simulink model "pendulum_demo"  (R2015a)
settings: Solver=ode45  SolverMode=SingleTasking  StartTime=0  StopTime=15  RelTol=1e-3  AbsTol=1e-6
PreLoadFcn:
  | load pendulum_demo
model workspace (MAT data in the model file):
  pendulum_optim = sldodialogs.data.SessionData
  pendulum_optim.Version = '3.0'
  pendulum_optim.Data.ModelName = 'pendulum_demo'
  pendulum_optim.Data.ToolData.ResponseOptimization.Options = sdo.OptimizeOptions
  pendulum_optim.Data.ToolData.ResponseOptimization.Options.Method = 'fminsearch'
  pendulum_optim.Data.ToolData.ResponseOptimization.Options.MethodOptions.Display = 'iter'
  pendulum_optim.Data.ToolData.ResponseOptimization.Options.MethodOptions.MaxFunEvals = 99
  pendulum_optim.Data.ToolData.ResponseOptimization.Options.MethodOptions.MaxIter = 49
  pendulum_optim.Data.ToolData.ResponseOptimization.Options.MethodOptions.TolFun = 0.001
  pendulum_optim.Data.ToolData.ResponseOptimization.Options.MethodOptions.TolX = 0.001
  pendulum_optim.Data.ToolData.ResponseOptimization.Options.MethodOptions.FunValCheck = 'off'
  pendulum_optim.Data.ToolData.ResponseOptimization.Options.MethodOptions.OutputFcn = []
  pendulum_optim.Data.ToolData.ResponseOptimization.Options.MethodOptions.PlotFcns = []
  pendulum_optim.Data.ToolData.ResponseOptimization.Options.MethodOptions.ActiveConstrTol = []
  pendulum_optim.Data.ToolData.ResponseOptimization.Options.MethodOptions.Algorithm = []
  pendulum_optim.Data.ToolData.ResponseOptimization.Options.MethodOptions.AlwaysHonorConstraints = []
  pendulum_optim.Data.ToolData.ResponseOptimization.Options.MethodOptions.BranchStrategy = []
  pendulum_optim.Data.ToolData.ResponseOptimization.Options.MethodOptions.DerivativeCheck = []
  pendulum_optim.Data.ToolData.ResponseOptimization.Options.MethodOptions.Diagnostics = []
  pendulum_optim.Data.ToolData.ResponseOptimization.Options.MethodOptions.DiffMaxChange = []
  pendulum_optim.Data.ToolData.ResponseOptimization.Options.MethodOptions.DiffMinChange = []
  pendulum_optim.Data.ToolData.ResponseOptimization.Options.MethodOptions.FinDiffRelStep = []
  pendulum_optim.Data.ToolData.ResponseOptimization.Options.MethodOptions.FinDiffType = []
  pendulum_optim.Data.ToolData.ResponseOptimization.Options.MethodOptions.GoalsExactAchieve = []
  pendulum_optim.Data.ToolData.ResponseOptimization.Options.MethodOptions.GradConstr = []
  pendulum_optim.Data.ToolData.ResponseOptimization.Options.MethodOptions.GradObj = []
  pendulum_optim.Data.ToolData.ResponseOptimization.Options.MethodOptions.HessFcn = []
  pendulum_optim.Data.ToolData.ResponseOptimization.Options.MethodOptions.Hessian = []
  pendulum_optim.Data.ToolData.ResponseOptimization.Options.MethodOptions.HessMult = []
  pendulum_optim.Data.ToolData.ResponseOptimization.Options.MethodOptions.HessPattern = []
  pendulum_optim.Data.ToolData.ResponseOptimization.Options.MethodOptions.HessUpdate = []
  pendulum_optim.Data.ToolData.ResponseOptimization.Options.MethodOptions.InitialHessType = []
  pendulum_optim.Data.ToolData.ResponseOptimization.Options.MethodOptions.InitialHessMatrix = []
  pendulum_optim.Data.ToolData.ResponseOptimization.Options.MethodOptions.InitBarrierParam = []
  pendulum_optim.Data.ToolData.ResponseOptimization.Options.MethodOptions.InitTrustRegionRadius = []
  pendulum_optim.Data.ToolData.ResponseOptimization.Options.MethodOptions.Jacobian = []
  pendulum_optim.Data.ToolData.ResponseOptimization.Options.MethodOptions.JacobMult = []
  pendulum_optim.Data.ToolData.ResponseOptimization.Options.MethodOptions.JacobPattern = []
  pendulum_optim.Data.ToolData.ResponseOptimization.Options.MethodOptions.LargeScale = []
  pendulum_optim.Data.ToolData.ResponseOptimization.Options.MethodOptions.LineSearchType = []
  pendulum_optim.Data.ToolData.ResponseOptimization.Options.MethodOptions.MaxNodes = []
  pendulum_optim.Data.ToolData.ResponseOptimization.Options.MethodOptions.MaxPCGIter = []
  pendulum_optim.Data.ToolData.ResponseOptimization.Options.MethodOptions.MaxProjCGIter = []
  pendulum_optim.Data.ToolData.ResponseOptimization.Options.MethodOptions.MaxRLPIter = []
  pendulum_optim.Data.ToolData.ResponseOptimization.Options.MethodOptions.MaxSQPIter = []
  pendulum_optim.Data.ToolData.ResponseOptimization.Options.MethodOptions.MaxTime = []
  pendulum_optim.Data.ToolData.ResponseOptimization.Options.MethodOptions.MeritFunction = []
  pendulum_optim.Data.ToolData.ResponseOptimization.Options.MethodOptions.MinAbsMax = []
  pendulum_optim.Data.ToolData.ResponseOptimization.Options.MethodOptions.NodeDisplayInterval = []
  pendulum_optim.Data.ToolData.ResponseOptimization.Options.MethodOptions.NodeSearchStrategy = []
  pendulum_optim.Data.ToolData.ResponseOptimization.Options.MethodOptions.NoStopIfFlatInfeas = []
  pendulum_optim.Data.ToolData.ResponseOptimization.Options.MethodOptions.ObjectiveLimit = []
  pendulum_optim.Data.ToolData.ResponseOptimization.Options.MethodOptions.PhaseOneTotalScaling = []
  pendulum_optim.Data.ToolData.ResponseOptimization.Options.MethodOptions.Preconditioner = []
  pendulum_optim.Data.ToolData.ResponseOptimization.Options.MethodOptions.PrecondBandWidth = []
  pendulum_optim.Data.ToolData.ResponseOptimization.Options.MethodOptions.RelLineSrchBnd = []
  pendulum_optim.Data.ToolData.ResponseOptimization.Options.MethodOptions.RelLineSrchBndDuration = []
  pendulum_optim.Data.ToolData.ResponseOptimization.Options.MethodOptions.ScaleProblem = []
  pendulum_optim.Data.ToolData.ResponseOptimization.Options.MethodOptions.Simplex = []
  pendulum_optim.Data.ToolData.ResponseOptimization.Options.MethodOptions.SubproblemAlgorithm = []
  pendulum_optim.Data.ToolData.ResponseOptimization.Options.MethodOptions.TolCon = 0.001
  pendulum_optim.Data.ToolData.ResponseOptimization.Options.MethodOptions.TolConSQP = []
  pendulum_optim.Data.ToolData.ResponseOptimization.Options.MethodOptions.TolGradCon = []
  pendulum_optim.Data.ToolData.ResponseOptimization.Options.MethodOptions.TolPCG = []
  pendulum_optim.Data.ToolData.ResponseOptimization.Options.MethodOptions.TolProjCG = []
  pendulum_optim.Data.ToolData.ResponseOptimization.Options.MethodOptions.TolProjCGAbs = []
  pendulum_optim.Data.ToolData.ResponseOptimization.Options.MethodOptions.TolRLPFun = []
  pendulum_optim.Data.ToolData.ResponseOptimization.Options.MethodOptions.TolXInteger = []
  pendulum_optim.Data.ToolData.ResponseOptimization.Options.MethodOptions.TypicalX = []
  pendulum_optim.Data.ToolData.ResponseOptimization.Options.MethodOptions.UseParallel = 'never'
  pendulum_optim.Data.ToolData.ResponseOptimization.DesignVariables = 'DesignVars'
  pendulum_optim.Data.ToolType = 'ResponseOptimization'
  pendulum_optim.Data.Workspace.LocalWorkspace.DesignVars(1) = param.Continuous
  pendulum_optim.Data.Workspace.LocalWorkspace.DesignVars(1).Scale_ = -3
  pendulum_optim.Data.Workspace.LocalWorkspace.DesignVars(1).Size_ = [1 1]
  pendulum_optim.Data.Workspace.LocalWorkspace.DesignVars(1).Value_ = -3
  pendulum_optim.Data.Workspace.LocalWorkspace.DesignVars(1).pID = paramid.Variable
  pendulum_optim.Data.Workspace.LocalWorkspace.DesignVars(1).pID.Name = 'Kf'
  pendulum_optim.Data.Workspace.LocalWorkspace.DesignVars(2) = param.Continuous
  pendulum_optim.Data.Workspace.LocalWorkspace.DesignVars(2).Scale_ = 0
  pendulum_optim.Data.Workspace.LocalWorkspace.DesignVars(2).Size_ = [1 1]
  pendulum_optim.Data.Workspace.LocalWorkspace.DesignVars(2).Value_ = 0
  pendulum_optim.Data.Workspace.LocalWorkspace.DesignVars(2).pID = paramid.Variable
  pendulum_optim.Data.Workspace.LocalWorkspace.DesignVars(2).pID.Name = 'Ki'
  pendulum_optim.Data.Workspace.LocalWorkspace.DesignVars(3) = param.Continuous
  pendulum_optim.Data.Workspace.LocalWorkspace.DesignVars(3).Scale_ = 4.81125224325
  pendulum_optim.Data.Workspace.LocalWorkspace.DesignVars(3).Size_ = [1 1]
  pendulum_optim.Data.Workspace.LocalWorkspace.DesignVars(3).Value_ = 4.81125224325
  pendulum_optim.Data.Workspace.LocalWorkspace.DesignVars(3).pID = paramid.Variable
  pendulum_optim.Data.Workspace.LocalWorkspace.DesignVars(3).pID.Name = 'Kp'
  pendulum_optim.Data.Workspace.HiddenWorkspace = []
undefined symbols (not defined in the file): Kf, Ki, Klqr, Kp
libraries: checkpacklib x2
settings Model: FPTRunName=Active  ExtModeTrigMode=oneshot  Creator=The MathWorks Inc.  LastModifiedBy=Panoply
settings DataIOCC: LimitDataPoints=off  SaveOutput=off  SaveTime=off  SignalLoggingName=logsOut
settings OptimizationCC: BooleanDataType=off  ExpressionDepthLimit=2147483647  InitFltsAndDblsToZero=on  EfficientMapNaN2IntZero=off
settings DebuggingCC: ConsistencyChecking=warning  SaveWithParameterizedLinksMsg=none  UnderspecifiedInitializationDetection=Classic  MergeDetectMultiDrivingBlocksExec=none  CheckExecutionContextPreStartOutputMsg=on  CheckExecutionContextRuntimeOutputMsg=on  SignalResolutionControl=TryResolveAllWithWarning  MultiTaskDSMMsg=warning  MultiTaskCondExecSysMsg=none  FcnCallInpInsideContextMsg=UseLocalSettings  StateNameClashWarn=warning
settings HardwareCC: TargetUnknown=on
settings ModelReferenceCC: UpdateModelReferenceTargets=IfOutOfDate
settings RTWCC: TemplateMakefile=grt_vc.tmf
settings GRTTargetCC: TargetFcnLib=ansi_tfl_tmw.mat  CombineOutputUpdateFcns=off  GRTInterface=on

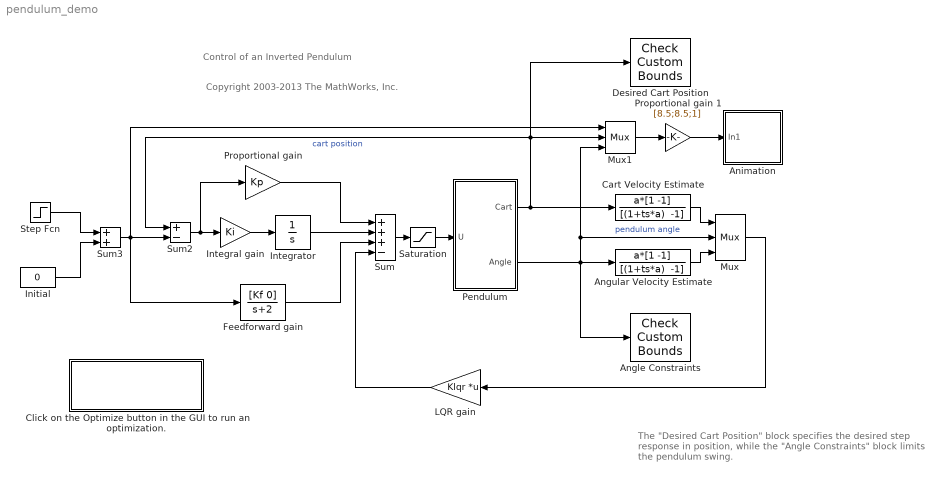
== system pendulum_demo ==
  note: Control of an Inverted Pendulum
  note: The "Desired Cart Position" block specifies the desired
      | step response in position, while the "Angle Constraints"
      | block limits the pendulum swing.
  note: Copyright 2003-2013 The MathWorks, Inc.
  Angle Constraints : checkpacklib/Check Custom Bounds  InstantiateOnLoad=on  enabled=on  stopWhenAssertionFail=off  export=off  ViewDlgPos=[541.717708333334 365.695 504.736979166666 296.7525]  OpenViewOnLoad=off  LaunchViewOnOpen=on  TimeUnits=seconds  EnableUpperBound=on  UpperBoundTimes=[0 15]  UpperBoundAmplitudes=[0.2 0.2]  EnableLowerBound=on  LowerBoundTimes=[0 15]  LowerBoundAmplitudes=[-0.2 -0.2]
  Angular Velocity Estimate : DiscreteTransferFcn  Numerator=a*[1 -1]  Denominator="[(1+ts*a)  -1]"  SampleTime=ts  mask(Finite difference velocity estimator with filter.){hz=10, ts=0.01}
      mask prompts: hz "Cutoff frequency( hz ):"; ts "Sample time:"
      mask help: Finite difference velocity estimator with filter.
      mask init:
      | a=hz*2*pi;
      mask Display: disp('FD w/ filter')
  Animation : Subsystem  mask(Pendulum plot){RefBlock=Initial, doAnimation=false}
      mask prompts: RefBlock "DC reference signal block name:"; doAnimation "Show animation"
      mask help: Pendulum plot
      mask Help: Pendulum animation function using Handle graphics.
      mask Display: plot([-10 10],[0 0],[-2 -2 2 2],[0 1 1 0],[0 3],[1 5])
  Cart Velocity Estimate : DiscreteTransferFcn  Numerator=a*[1 -1]  Denominator="[(1+ts*a)  -1]"  SampleTime=ts  mask(Finite difference velocity estimator with filter.){hz=10, ts=0.01}
      mask prompts: hz "Cutoff frequency( hz ):"; ts "Sample time:"
      mask help: Finite difference velocity estimator with filter.
      mask init:
      | a=hz*2*pi;
      mask Display: disp('FD w/ filter')
  Click on the Optimize button in the GUI to run an optimization. : Subsystem
      settings: OpenFcn=sdotool( slResolve('pendulum_optim', 'pendulum_demo') );
      mask Display: disp('Response Optimization\nGUI with preloaded data')
  Desired Cart Position : checkpacklib/Check Custom Bounds  InstantiateOnLoad=on  enabled=on  stopWhenAssertionFail=off  export=off  ViewDlgPos=[262 234 511 298]  OpenViewOnLoad=on  LaunchViewOnOpen=on  TimeUnits=seconds  EnableUpperBound=on  UpperBoundTimes=[0 6;6 15]  UpperBoundAmplitudes=[1.1 1.1;1.01 1.01]  EnableLowerBound=on  LowerBoundTimes=[0 3;3 6;6 15]  LowerBoundAmplitudes=[-0.1 -0.1;0.882608695652174 0.882608695652174;0.99 0.99]
  Feedforward gain : TransferFcn  Numerator=[Kf 0]  Denominator=[1 2]
  Initial : Constant  Value=0
  Integral gain : Gain  Gain=Ki  SaturateOnIntegerOverflow=on  OutDataTypeStr=Inherit: Same as input  ParamDataTypeStr=Inherit: Same as input
  Integrator : Integrator  LimitOutput=on  UpperSaturationLimit=5  LowerSaturationLimit=-5
  LQR gain : Gain  Gain=Klqr  Multiplication=Matrix(K*u)
  Mux : Mux  Inputs=3
  Mux1 : Mux  Inputs=3
  Pendulum : Subsystem  mask(Inverted pendulum on cart){Mcart=0.455, m=0.21, l=0.61/2, g=9.8}
      mask prompts: Mcart "Mass of cart (kg):"; m "Mass of pendulum (kg):"; l "Distance to pendulum center of mass(m):"; g "Acceleration of gravity (m/s^2):"
      mask help: Unmask and double-click to see dynamics
      mask Help: Nonlinear dynamics of inverted pendulum on cart.
  "Proportional gain " : Gain  Gain=Kp  SaturateOnIntegerOverflow=on  OutDataTypeStr=Inherit: Same as input  ParamDataTypeStr=Inherit: Same as input
  Proportional gain 1 : Gain  Gain=[8.5;8.5;1]  SaturateOnIntegerOverflow=on  OutDataTypeStr=Inherit: Same as input  ParamDataTypeStr=Inherit: Same as input
  Saturation : Saturate  UpperLimit=1  LowerLimit=-1
  Step Fcn : Step  Time=0  SampleTime=0
  Sum : Sum  Inputs=+++-  SaturateOnIntegerOverflow=on  InputSameDT=on  OutDataTypeStr=Inherit: Same as first input
  Sum2 : Sum  Inputs=+-  SaturateOnIntegerOverflow=on  InputSameDT=on  OutDataTypeStr=Inherit: Same as first input
  Sum3 : Sum  SaturateOnIntegerOverflow=on  InputSameDT=on  OutDataTypeStr=Inherit: Same as first input
  wires:
  Mux/1 -> LQR gain/1
  LQR gain/1 -> Sum/4
  Sum2/1 -> Integral gain/1, "Proportional gain "/1
  Integral gain/1 -> Integrator/1
  Sum/1 -> Saturation/1
  "Proportional gain "/1 -> Sum/1
  Feedforward gain/1 -> Sum/3
  Sum3/1 -> Feedforward gain/1, Sum2/2, Mux1/1
  Integrator/1 -> Sum/2
  Saturation/1 -> Pendulum/1(U)
  Pendulum/1(Cart) -> Sum2/1, Desired Cart Position/1, Mux1/2, Cart Velocity Estimate/1  "cart position"
  Cart Velocity Estimate/1 -> Mux/1
  Angular Velocity Estimate/1 -> Mux/3
  Mux1/1 -> Proportional gain 1/1
  Initial/1 -> Sum3/2
  Step Fcn/1 -> Sum3/1
  Pendulum/2(Angle) -> Angular Velocity Estimate/1, Angle Constraints/1, Mux1/3, Mux/2  "pendulum angle"
  Proportional gain 1/1 -> Animation/1(In1)

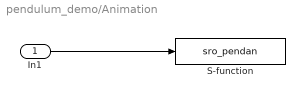
== system pendulum_demo/Animation ==
  In1 : Inport
  S-function : S-Function  FunctionName=sro_pendan  Parameters=RefBlock, doAnimation
      settings: DeleteFcn=sro_pendan([],[],[],'DeleteBlock');
  wires:
  In1/1 -> S-function/1

== system pendulum_demo/Click on the Optimize button in the GUI to run an optimization. ==

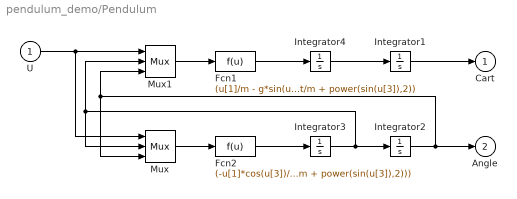
== system pendulum_demo/Pendulum ==
  U : Inport
  Fcn1 : Fcn  Expr=(u[1]/m - g*sin(u[3])*cos(u[3]) + l*power(u[2],2)*sin(u[3]))/(Mcart/m + power(sin(u[3]),2))
  Fcn2 : Fcn  Expr=(-u[1]*cos(u[3])/m + (Mcart+m)*g*sin(u[3])/m - l*power(u[2],2)*sin(u[3])*cos(u[3]))/(l*(Mcart/m + power(sin(u[3]),2)))
  Integrator{1..4} (4 alike) : Integrator
  Mux : Mux  Inputs=3
  Mux1 : Mux  Inputs=3
  Cart : Outport  InitialOutput=0
  Angle : Outport  Port=2  InitialOutput=0
  wires:
  Integrator2/1 -> Mux/3, Mux1/3, Angle/1
  Integrator3/1 -> Mux/2, Mux1/2, Integrator2/1
  U/1 -> Mux/1, Mux1/1
  Integrator4/1 -> Integrator1/1
  Fcn1/1 -> Integrator4/1
  Mux1/1 -> Fcn1/1
  Mux/1 -> Fcn2/1
  Fcn2/1 -> Integrator3/1
  Integrator1/1 -> Cart/1
